simulink model "Astrom_8_4"  (Simulink 6.6)
settings: Solver=ode45  StartTime=0.0  StopTime=10.0  RelTol=1e-3
values from neighbouring files (symbols this model uses):
  h = findobj(gcf,'type','line')    [boldLines.m]    (also in phase.m = min(hmax, 0.9*h*(tau/delta)^pow))
settings Model: Creator=Michael Sebek  ModifiedByFormat=Michael Sebek  LastModifiedBy=Michael Sebek
settings DebuggingCC: SignalResolutionControl=TryResolveAllWithWarning  MultiTaskDSMMsg=warning  MultiTaskCondExecSysMsg=none  StrictBusMsg=None
settings RTWCC: IncludeERTFirstTime=on

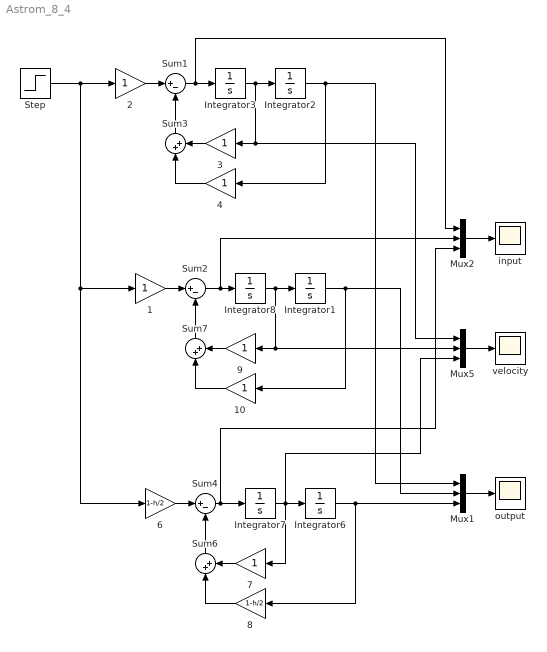
== system Astrom_8_4 ==
  1 : Gain
  10 : Gain  Orientation=left  SampleTime=h
  2 : Gain
  3 : Gain  Orientation=left
  4 : Gain  Orientation=left
  6 : Gain  Gain=1-h/2
  7 : Gain  Orientation=left  SampleTime=h
  8 : Gain  Orientation=left  Gain=1-h/2  SampleTime=h
  9 : Gain  Orientation=left  SampleTime=h
  Integrator{1..3,6..8} (6 alike) : Integrator
  Mux1 : Mux  Inputs=3
  Mux2 : Mux  Inputs=3
  Mux5 : Mux  Inputs=3
  Step : Step  Time=0  SampleTime=0
  Sum1 : Sum  Inputs=|+-
  Sum2 : Sum  Inputs=|+-
  Sum3 : Sum  Orientation=up  Inputs=|++
  Sum4 : Sum  Inputs=|+-
  Sum6 : Sum  Orientation=up  Inputs=|++
  Sum7 : Sum  Orientation=up  Inputs=|++
  input : Scope
  output : Scope
  velocity : Scope
      settings: SaveName=ScopeData5
  wires:
  Step/1 -> 2/1, 1/1, 6/1
  Integrator2/1 -> 4/1, Mux1/1
  Sum1/1 -> Integrator3/1, Mux2/1
  2/1 -> Sum1/1
  Integrator3/1 -> Integrator2/1, 3/1, Mux5/1
  Sum3/1 -> Sum1/2
  4/1 -> Sum3/1
  3/1 -> Sum3/2
  Integrator6/1 -> 8/1, Mux1/3
  Sum4/1 -> Integrator7/1, Mux2/3
  6/1 -> Sum4/1
  Integrator7/1 -> Integrator6/1, 7/1, Mux5/3
  Mux5/1 -> velocity/1
  Sum6/1 -> Sum4/2
  8/1 -> Sum6/1
  7/1 -> Sum6/2
  Integrator1/1 -> 10/1, Mux1/2
  Sum2/1 -> Integrator8/1, Mux2/2
  1/1 -> Sum2/1
  Integrator8/1 -> Integrator1/1, 9/1, Mux5/2
  Sum7/1 -> Sum2/2
  10/1 -> Sum7/1
  9/1 -> Sum7/2
  Mux1/1 -> output/1
  Mux2/1 -> input/1
